simulink model "digital_filter_resample"  (R2015b)
settings: Solver=VariableStepAuto  StartTime=0.0  StopTime=10.0  RelTol=1e-3
values from neighbouring files (symbols this model uses):
  a = -1    [abs_spring18.m]    (also in hw_tank_simulink_pid_tuning.m = 2.085; pmsm_fall19.m = 0.427011494253; rhszero_variables.m = 4; tanker_yaw_lead_zero.m)
  b = [0.6-1.84; 0.18-1; 0]    [final_dummy.m]    (also in pmsm_fall19.m = 4024.13793103)
libraries: simulink x1
settings Model: Creator=kjartan  LastModifiedBy=kjartan

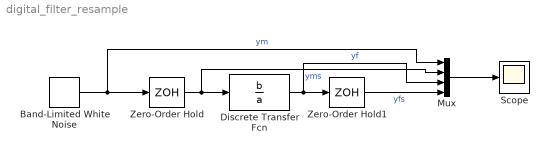
== system digital_filter_resample ==
  Band-Limited White Noise : simulink/Sources/Band-Limited White Noise  Cov=1  Ts=0.001  seed=[23341]
  Discrete Transfer Fcn : DiscreteTransferFcn  Numerator=b  Denominator=a  SampleTime=0.001
  Mux : Mux
  Scope : Scope
  Zero-Order Hold : ZeroOrderHold  SampleTime=0.001
  Zero-Order Hold1 : ZeroOrderHold  SampleTime=0.1
  wires:
  Band-Limited White Noise/1 -> Mux/1, Zero-Order Hold/1  "ym"
  Zero-Order Hold/1 -> Mux/2, Discrete Transfer Fcn/1  "yms"
  Discrete Transfer Fcn/1 -> Mux/3, Zero-Order Hold1/1  "yf"
  Zero-Order Hold1/1 -> Mux/4  "yfs"
  Mux/1 -> Scope/1
